simulink model "North_Country_Grid_2024a"  (R2024a)
settings: Solver=VariableStepAuto  StartTime=0.0  StopTime=10  RelTol=1e-3
PreLoadFcn:
  | Ts=50e-6;
InitFcn:
  | xInitial = WindFarmType4AverageModelInit;
  | Ts=50e-6;
undefined symbols (not defined in the file or in its folder): D1, D11, Delta, DiscIntNeverNeededParam, find_system, Fnom_I, Fnom_R, Idc_nom, lagging, level, pulse, test_alpha, Vdc_nom, VLL_nom_I, VLL_nom_R
libraries: spsSecondOrderFilterLib x47, powerlib_extras x38, simulink x34, spsThreePhaseVIMeasurementLib x30, spsFirstOrderFilterLib x29, simulink_extras x26, spsabctodq0Lib x25, spsThreePhaseTransformerTwoWindingsLib x19, spsThreePhaseBreakerLib x18, spsThreePhasePISectionLineLib x17, spsControlledVoltageSourceLib x15, spsOnDelayLib x12
(part 7 of 18)

== system North_Country_Grid_2024a/Noble Chateauguay (Type 4, 106.5 MW)/Wind Farm/Inverter and DC-DC Converter Average Models ==
  note: Pac=Vab*Ia -Vbc*Ic
      | Pdc=Vdc*Idc
  note: Vab Vbc Inverter
      | Average Model
  note: DC-DC Converter
      | Average Model
  note: Inverter and DC-DC Boost Converter
      | Average Models
  note: Current of the boost converter diode
      | This diode is not illustrated in the average model
  IL : Inport
  Iabc_grid_conv : Inport  Port=2
  Uctrl_inverter : Inport  Port=3
  Duty_Cycle : Inport  Port=4
  0.1 : Gain  Gain=0.5
  0.2 : Gain  Gain=-1
  0.5 : Gain  Gain=0.5
  1/C : Gain  Gain=1/C_DClink
  Constant2 : Constant
  Demux : Demux  Outputs=3
  Demux2 : Demux  Outputs=3
  Discrete-Time Integrator : DiscreteIntegrator  InitialCondition=Vdc_nom  SampleTime=Ts  LimitOutput=on  LowerSaturationLimit=eps  ICPrevOutput=DiscIntNeverNeededParam  ICPrevScaledInput=DiscIntNeverNeededParam
  Product{1..4,6..7} (6 alike) : Product  RndMeth=Zero
  Product5 : Product  Inputs=*/  RndMeth=Zero
  Saturation Dynamic : simulink/Discontinuities/Saturation Dynamic  OutMin=[]  OutMax=[]  OutDataTypeStr=Inherit: Same as second input  OutDataType=sfix(16)  OutScaling=2^-10  DoSatur=off
  Saturation Dynamic1 : simulink/Discontinuities/Saturation Dynamic  OutMin=[]  OutMax=[]  OutDataTypeStr=Inherit: Same as second input  OutDataType=sfix(16)  OutScaling=2^-10  DoSatur=off
  Subtract1 : Sum  Inputs=+-
  Subtract2 : Sum  Inputs=+-
  Subtract3 : Sum  Inputs=+-
  Subtract4 : Sum
  Sum : Sum  Inputs=|+-
  Terminator : Terminator
  pu->A : Gain  Gain=Pnom/(3*sqrt(2)/pi*Vnom_gen)  SaturateOnIntegerOverflow=on  OutDataTypeStr=Inherit: Same as input  ParamDataTypeStr=Inherit: Same as input
  "pu->A " : Gain  Gain=Pnom/sqrt(3)/Vnom*sqrt(2)  SaturateOnIntegerOverflow=on  OutDataTypeStr=Inherit: Same as input  ParamDataTypeStr=Inherit: Same as input
  Vab (V) : Outport  VectorParamsAs1DForOutWhenUnconnected=off
  Vbc (V) : Outport  Port=2  VectorParamsAs1DForOutWhenUnconnected=off
  Vswitch (V) : Outport  Port=3  VectorParamsAs1DForOutWhenUnconnected=off
  Vdc (V) : Outport  Port=4  VectorParamsAs1DForOutWhenUnconnected=off
  wires:
  Product1/1 -> Vswitch (V)/1
  Product2/1 -> [Idiode]
  [Vdc] -> Product1/1
  IL/1 -> pu->A/1
  Sum/1 -> Product2/1, Product1/2
  Constant2/1 -> Sum/1
  1/C/1 -> Discrete-Time Integrator/1
  Discrete-Time Integrator/1 -> Vdc (V)/1, Product5/2, [Vdc]
  Subtract4/1 -> 1/C/1
  Demux/1 -> Product3/2  "Ia"
  "pu->A "/1 -> Demux/1
  Demux/2 -> Terminator/1
  Iabc_grid_conv/1 -> "pu->A "/1
  Duty_Cycle/1 -> Sum/2
  Product4/1 -> Subtract2/2
  Product3/1 -> Subtract2/1
  Subtract2/1 -> Product5/1  "Pac"
  Demux/3 -> Product4/2  "Ic"
  [Vab] -> Product3/1
  [Vbc] -> Product4/1
  Product5/1 -> Subtract4/2  "Idc grid converter"
  [Vdc] -> 0.2/1, Saturation Dynamic1/1, Saturation Dynamic/1, Product6/2, Product7/2
  Subtract1/1 -> Product7/1
  Subtract3/1 -> Product6/1
  Product7/1 -> 0.1/1
  Product6/1 -> 0.5/1
  Demux2/3 -> Subtract1/2
  Demux2/2 -> Subtract3/2, Subtract1/1
  Demux2/1 -> Subtract3/1
  0.5/1 -> Saturation Dynamic/2  "Vab_avg"
  0.1/1 -> Saturation Dynamic1/2  "Vbc_avg"
  0.2/1 -> Saturation Dynamic/3, Saturation Dynamic1/3
  Uctrl_inverter/1 -> Demux2/1
  Saturation Dynamic/1 -> Vab (V)/1, [Vab]
  Saturation Dynamic1/1 -> Vbc (V)/1, [Vbc]
  [Idiode] -> Subtract4/1  "Idiode"
  pu->A/1 -> Product2/2

== system North_Country_Grid_2024a/Noble Chateauguay (Type 4, 106.5 MW)/Wind Farm/Wind Turbine ==
  W_wt (pu) : Inport
  Pitch angle (deg) : Inport  Port=2
  Wind speed (m/s) : Inport  Port=3
  ->pu : Gain  Gain=1/Prated
  Avoid div. by zero : Saturate  UpperLimit=inf  LowerLimit=eps
  "Avoid div. by zero " : Saturate  UpperLimit=inf  LowerLimit=eps
  Fcn1 : Fcn  Expr=K1*u[2]/u[1]
  Fcn2 : Fcn  Expr=c1*(c6*u[1] + (-c4 - c3*(2.5 + u[2]) + c2*(1/(u[1] + c7*(2.5 + u[2])) -c8/(1 + (2.5 + u[2])^3)))/exp(c5*(1/(u[1] + c7*(2.5 + u[2])) - c8/(1 + (2.5 + u[2])^3))))
  "K2*Cp*wind^3 " : Fcn  Expr=K2*u[1]^3*u[2]
  Mux : Mux  Inputs=2
  Mux1 : Mux  Inputs=2
  Mux2 : Mux  Inputs=2
  Product2 : Product  Inputs=*/  InputSameDT=on  SaturateOnIntegerOverflow=on  OutDataTypeStr=Inherit: Same as first input
  Tt (pu) : Outport  VectorParamsAs1DForOutWhenUnconnected=off
  wires:
  ->pu/1 -> Product2/1  "power_pu"
  Product2/1 -> Tt (pu)/1
  Wind speed (m/s)/1 -> Avoid div. by zero/1
  Fcn1/1 -> Mux1/1  "lambda"
  Mux1/1 -> Fcn2/1
  Mux/1 -> Fcn1/1
  Fcn2/1 -> Mux2/2  "Cp"
  Mux2/1 -> "K2*Cp*wind^3 "/1
  Pitch angle (deg)/1 -> Mux1/2
  W_wt (pu)/1 -> "Avoid div. by zero "/1
  Avoid div. by zero/1 -> Mux2/1, Mux/1
  "Avoid div. by zero "/1 -> Mux/2, Product2/2
  "K2*Cp*wind^3 "/1 -> ->pu/1

== system North_Country_Grid_2024a/Noble Clinton (Type 4, 100.5 MW)/Wind Farm/Average Switch Voltage ==
  Vswitch : Inport
  Diode : spsDiodeLib/Diode  Ron=1e-6/Nb_wt  Lon=0  Vf=0  IC=0  UseSnubber=off  Rs=1e5  Cs=inf  Measurements=off
  V : spsControlledVoltageSourceLib/Controlled Voltage Source  Initialize=on  Source_Type=AC  Amplitude=0  Phase=0  Frequency=0  Measurements=None
  + : PMIOPort  Side=Right
  - : PMIOPort  Port=2  Side=Left
  wires:
  Vswitch/1 -> V/1
  connections:
  Diode/RConn1 -- V/RConn1
  +/RConn1 -- Diode/LConn1
  -/RConn1 -- V/LConn1

== system North_Country_Grid_2024a/Noble Clinton (Type 4, 100.5 MW)/Wind Farm/Control ==
  note: Inputs
  note: Grid-Side Converter
      | Control System
  note: Speed Regulator & Pitch Control
  note: Excitation
      | Control system
  Vabc_grid : Inport
  Iabc_grid_conv : Inport  Port=2
  Vabc_LL_stator : Inport  Port=3
  Iabc_stator : Inport  Port=4
  IL : Inport  Port=5
  Vdc : Inport  Port=6
  Qref : Inport  Port=7
  angle_rotor : Inport  Port=8
  wr : Inport  Port=9
  Bus Creator : BusCreator  Inputs=2
  Excitation Control system : Subsystem
  Grid-side converter Control system : Subsystem
  Measurement and Transformation : Subsystem
  Speed & Pitch Control : Subsystem
  Unit Delay{1..4,6..7} (6 alike) : UnitDelay  SampleTime=Ts  HasFrameUpgradeWarning=on
  Uctrl_inverter : Outport  VectorParamsAs1DForOutWhenUnconnected=off
  Duty_Cycle : Outport  Port=2  VectorParamsAs1DForOutWhenUnconnected=off
  Pitch_angle : Outport  Port=3  VectorParamsAs1DForOutWhenUnconnected=off
  Vf : Outport  Port=4  VectorParamsAs1DForOutWhenUnconnected=off
  PQ_pu : Outport  Port=5  VectorParamsAs1DForOutWhenUnconnected=off
  wires:
  Excitation Control system/1(Vf) -> Unit Delay2/1
  Speed & Pitch Control/2(Pitch (deg)) -> Unit Delay4/1
  Measurement and Transformation/7(Qmeas) -> [Qmeas]
  Measurement and Transformation/1(Vdq_grid) -> [Vdq_grid]
  Measurement and Transformation/2(Idq_gc) -> [Idq_gc]
  Measurement and Transformation/6(Pmeas) -> [Pmeas]
  Measurement and Transformation/8(Vmeas) -> [Vmeas]
  Measurement and Transformation/10(w_pu) -> [w_pu]
  [Idq_gc] -> Grid-side converter Control system/1(Idq_gc)
  [w_pu] -> Grid-side converter Control system/2(w_pu)
  [Vdq_grid] -> Grid-side converter Control system/3(Vdq_grid)
  [Vdc_meas] -> Grid-side converter Control system/4(Vdc)
  Measurement and Transformation/5(Vdc_meas) -> [Vdc_meas]
  Measurement and Transformation/11("wr ") -> [wr]
  Measurement and Transformation/12("Qref ") -> [Qref]
  [Qref] -> Grid-side converter Control system/5(Qref)
  [Qmeas] -> Grid-side converter Control system/6(Qmeas)
  [Vmeas] -> Grid-side converter Control system/7(Vmeas)
  [wr] -> Speed & Pitch Control/1(wr)
  [Pmeas] -> Speed & Pitch Control/2(Pmeas)
  Speed & Pitch Control/1(Duty_Cycle) -> Unit Delay1/1
  Measurement and Transformation/4(Flux) -> [Flux]
  [Flux] -> Excitation Control system/1(Flux)
  [wr] -> Excitation Control system/2(wr)
  Vabc_grid/1 -> Measurement and Transformation/1(Vabc_grid)
  Iabc_grid_conv/1 -> Measurement and Transformation/2(Iabc_gc)
  Vabc_LL_stator/1 -> Measurement and Transformation/3(Vabc_LL_s)
  Iabc_stator/1 -> Measurement and Transformation/4(Iabc_s)
  Vdc/1 -> Measurement and Transformation/6(Vdc)
  Qref/1 -> Measurement and Transformation/7(Qref)
  angle_rotor/1 -> Measurement and Transformation/8(angle_rotor)
  wr/1 -> Measurement and Transformation/9(wr)
  Grid-side converter Control system/1(Uctrl_inverter) -> Unit Delay3/1
  [Theta_PLL] -> Grid-side converter Control system/8(Theta_PLL)
  Measurement and Transformation/9(Theta_PLL) -> [Theta_PLL]
  Bus Creator/1 -> PQ_pu/1
  Unit Delay3/1 -> Uctrl_inverter/1
  Unit Delay2/1 -> Vf/1
  Unit Delay1/1 -> Duty_Cycle/1
  Unit Delay4/1 -> Pitch_angle/1
  [Pmeas] -> Unit Delay6/1
  [Qmeas] -> Unit Delay7/1
  Unit Delay6/1 -> Bus Creator/1  "P_pu"
  Unit Delay7/1 -> Bus Creator/2  "Q_pu"
  Measurement and Transformation/3("IL ") -> [IL]
  IL/1 -> Measurement and Transformation/5(IL)
  [IL] -> Speed & Pitch Control/3(IL)

== system North_Country_Grid_2024a/Noble Clinton (Type 4, 100.5 MW)/Wind Farm/Drive Train ==
  note: Wind turbine drive train based on a 2-masse model
  note: Turbine
  note: Shaft
  T_wt (pu) : Inport
  Generator speed (pu) : Inport  Port=2
  1_2H_WT : Gain  Gain=1/(2*H_WT)  SaturateOnIntegerOverflow=on  OutDataTypeStr=Inherit: Same as input  ParamDataTypeStr=Inherit: Same as input
  Discrete-Time Integrator : DiscreteIntegrator  InitialCondition=w_wt0  SampleTime=Ts  ICPrevOutput=DiscIntNeverNeededParam  ICPrevScaledInput=DiscIntNeverNeededParam
  Discrete-Time Integrator1 : DiscreteIntegrator  InitialCondition=torque0/Ksh  SampleTime=Ts  ICPrevOutput=DiscIntNeverNeededParam  ICPrevScaledInput=DiscIntNeverNeededParam
  Mutual damping : Gain  Gain=D_mutual  SaturateOnIntegerOverflow=on  OutDataTypeStr=Inherit: Same as input  ParamDataTypeStr=Inherit: Same as input
  Stiffness : Gain  Gain=Ksh  SaturateOnIntegerOverflow=on  OutDataTypeStr=Inherit: Same as input  ParamDataTypeStr=Inherit: Same as input
  Sum : Sum  Inputs=+-  InputSameDT=on  SaturateOnIntegerOverflow=on  OutDataTypeStr=Inherit: Same as first input
  Sum1 : Sum  Inputs=+-  InputSameDT=on  SaturateOnIntegerOverflow=on  OutDataTypeStr=Inherit: Same as first input
  Sum2 : Sum  InputSameDT=on  SaturateOnIntegerOverflow=on  OutDataTypeStr=Inherit: Same as first input
  wbase : Gain  Gain=wbase  SaturateOnIntegerOverflow=on  OutDataTypeStr=Inherit: Same as input  ParamDataTypeStr=Inherit: Same as input
  W_wt (pu) : Outport  VectorParamsAs1DForOutWhenUnconnected=off
  T_shaft (pu) : Outport  Port=2  VectorParamsAs1DForOutWhenUnconnected=off
  wires:
  T_wt (pu)/1 -> Sum/1
  Sum2/1 -> T_shaft (pu)/1, Sum/2
  Mutual damping/1 -> Sum2/2
  Sum1/1 -> Mutual damping/1, wbase/1
  Generator speed (pu)/1 -> Sum1/2
  Discrete-Time Integrator/1 -> W_wt (pu)/1, Sum1/1
  1_2H_WT/1 -> Discrete-Time Integrator/1
  Sum/1 -> 1_2H_WT/1
  Stiffness/1 -> Sum2/1
  Discrete-Time Integrator1/1 -> Stiffness/1
  wbase/1 -> Discrete-Time Integrator1/1

== system North_Country_Grid_2024a/Noble Clinton (Type 4, 100.5 MW)/Wind Farm/Inverter and DC-DC Converter Average Models ==
  note: Pac=Vab*Ia -Vbc*Ic
      | Pdc=Vdc*Idc
  note: Vab Vbc Inverter
      | Average Model
  note: DC-DC Converter
      | Average Model
  note: Inverter and DC-DC Boost Converter
      | Average Models
  note: Current of the boost converter diode
      | This diode is not illustrated in the average model
  IL : Inport
  Iabc_grid_conv : Inport  Port=2
  Uctrl_inverter : Inport  Port=3
  Duty_Cycle : Inport  Port=4
  0.1 : Gain  Gain=0.5
  0.2 : Gain  Gain=-1
  0.5 : Gain  Gain=0.5
  1/C : Gain  Gain=1/C_DClink
  Constant2 : Constant
  Demux : Demux  Outputs=3
  Demux2 : Demux  Outputs=3
  Discrete-Time Integrator : DiscreteIntegrator  InitialCondition=Vdc_nom  SampleTime=Ts  LimitOutput=on  LowerSaturationLimit=eps  ICPrevOutput=DiscIntNeverNeededParam  ICPrevScaledInput=DiscIntNeverNeededParam
  Product{1..4,6..7} (6 alike) : Product  RndMeth=Zero
  Product5 : Product  Inputs=*/  RndMeth=Zero
  Saturation Dynamic : simulink/Discontinuities/Saturation Dynamic  OutMin=[]  OutMax=[]  OutDataTypeStr=Inherit: Same as second input  OutDataType=sfix(16)  OutScaling=2^-10  DoSatur=off
  Saturation Dynamic1 : simulink/Discontinuities/Saturation Dynamic  OutMin=[]  OutMax=[]  OutDataTypeStr=Inherit: Same as second input  OutDataType=sfix(16)  OutScaling=2^-10  DoSatur=off
  Subtract1 : Sum  Inputs=+-
  Subtract2 : Sum  Inputs=+-
  Subtract3 : Sum  Inputs=+-
  Subtract4 : Sum
  Sum : Sum  Inputs=|+-
  Terminator : Terminator
  pu->A : Gain  Gain=Pnom/(3*sqrt(2)/pi*Vnom_gen)  SaturateOnIntegerOverflow=on  OutDataTypeStr=Inherit: Same as input  ParamDataTypeStr=Inherit: Same as input
  "pu->A " : Gain  Gain=Pnom/sqrt(3)/Vnom*sqrt(2)  SaturateOnIntegerOverflow=on  OutDataTypeStr=Inherit: Same as input  ParamDataTypeStr=Inherit: Same as input
  Vab (V) : Outport  VectorParamsAs1DForOutWhenUnconnected=off
  Vbc (V) : Outport  Port=2  VectorParamsAs1DForOutWhenUnconnected=off
  Vswitch (V) : Outport  Port=3  VectorParamsAs1DForOutWhenUnconnected=off
  Vdc (V) : Outport  Port=4  VectorParamsAs1DForOutWhenUnconnected=off
  wires:
  Product1/1 -> Vswitch (V)/1
  Product2/1 -> [Idiode]
  [Vdc] -> Product1/1
  IL/1 -> pu->A/1
  Sum/1 -> Product2/1, Product1/2
  Constant2/1 -> Sum/1
  1/C/1 -> Discrete-Time Integrator/1
  Discrete-Time Integrator/1 -> Vdc (V)/1, Product5/2, [Vdc]
  Subtract4/1 -> 1/C/1
  Demux/1 -> Product3/2  "Ia"
  "pu->A "/1 -> Demux/1
  Demux/2 -> Terminator/1
  Iabc_grid_conv/1 -> "pu->A "/1
  Duty_Cycle/1 -> Sum/2
  Product4/1 -> Subtract2/2
  Product3/1 -> Subtract2/1
  Subtract2/1 -> Product5/1  "Pac"
  Demux/3 -> Product4/2  "Ic"
  [Vab] -> Product3/1
  [Vbc] -> Product4/1
  Product5/1 -> Subtract4/2  "Idc grid converter"
  [Vdc] -> 0.2/1, Saturation Dynamic1/1, Saturation Dynamic/1, Product6/2, Product7/2
  Subtract1/1 -> Product7/1
  Subtract3/1 -> Product6/1
  Product7/1 -> 0.1/1
  Product6/1 -> 0.5/1
  Demux2/3 -> Subtract1/2
  Demux2/2 -> Subtract3/2, Subtract1/1
  Demux2/1 -> Subtract3/1
  0.5/1 -> Saturation Dynamic/2  "Vab_avg"
  0.1/1 -> Saturation Dynamic1/2  "Vbc_avg"
  0.2/1 -> Saturation Dynamic/3, Saturation Dynamic1/3
  Uctrl_inverter/1 -> Demux2/1
  Saturation Dynamic/1 -> Vab (V)/1, [Vab]
  Saturation Dynamic1/1 -> Vbc (V)/1, [Vbc]
  [Idiode] -> Subtract4/1  "Idiode"
  pu->A/1 -> Product2/2

== system North_Country_Grid_2024a/Noble Clinton (Type 4, 100.5 MW)/Wind Farm/Wind Turbine ==
  W_wt (pu) : Inport
  Pitch angle (deg) : Inport  Port=2
  Wind speed (m/s) : Inport  Port=3
  ->pu : Gain  Gain=1/Prated
  Avoid div. by zero : Saturate  UpperLimit=inf  LowerLimit=eps
  "Avoid div. by zero " : Saturate  UpperLimit=inf  LowerLimit=eps
  Fcn1 : Fcn  Expr=K1*u[2]/u[1]
  Fcn2 : Fcn  Expr=c1*(c6*u[1] + (-c4 - c3*(2.5 + u[2]) + c2*(1/(u[1] + c7*(2.5 + u[2])) -c8/(1 + (2.5 + u[2])^3)))/exp(c5*(1/(u[1] + c7*(2.5 + u[2])) - c8/(1 + (2.5 + u[2])^3))))
  "K2*Cp*wind^3 " : Fcn  Expr=K2*u[1]^3*u[2]
  Mux : Mux  Inputs=2
  Mux1 : Mux  Inputs=2
  Mux2 : Mux  Inputs=2
  Product2 : Product  Inputs=*/  InputSameDT=on  SaturateOnIntegerOverflow=on  OutDataTypeStr=Inherit: Same as first input
  Tt (pu) : Outport  VectorParamsAs1DForOutWhenUnconnected=off
  wires:
  ->pu/1 -> Product2/1  "power_pu"
  Product2/1 -> Tt (pu)/1
  Wind speed (m/s)/1 -> Avoid div. by zero/1
  Fcn1/1 -> Mux1/1  "lambda"
  Mux1/1 -> Fcn2/1
  Mux/1 -> Fcn1/1
  Fcn2/1 -> Mux2/2  "Cp"
  Mux2/1 -> "K2*Cp*wind^3 "/1
  Pitch angle (deg)/1 -> Mux1/2
  W_wt (pu)/1 -> "Avoid div. by zero "/1
  Avoid div. by zero/1 -> Mux2/1, Mux/1
  "Avoid div. by zero "/1 -> Mux/2, Product2/2
  "K2*Cp*wind^3 "/1 -> ->pu/1

== system North_Country_Grid_2024a/Noble Ellenburg (Type 4, 81 MW)/Wind Farm/Average Switch Voltage ==
  Vswitch : Inport
  Diode : spsDiodeLib/Diode  Ron=1e-6/Nb_wt  Lon=0  Vf=0  IC=0  UseSnubber=off  Rs=1e5  Cs=inf  Measurements=off
  V : spsControlledVoltageSourceLib/Controlled Voltage Source  Initialize=on  Source_Type=AC  Amplitude=0  Phase=0  Frequency=0  Measurements=None
  + : PMIOPort  Side=Right
  - : PMIOPort  Port=2  Side=Left
  wires:
  Vswitch/1 -> V/1
  connections:
  Diode/RConn1 -- V/RConn1
  +/RConn1 -- Diode/LConn1
  -/RConn1 -- V/LConn1

== system North_Country_Grid_2024a/Noble Ellenburg (Type 4, 81 MW)/Wind Farm/Control ==
  note: Inputs
  note: Grid-Side Converter
      | Control System
  note: Speed Regulator & Pitch Control
  note: Excitation
      | Control system
  Vabc_grid : Inport
  Iabc_grid_conv : Inport  Port=2
  Vabc_LL_stator : Inport  Port=3
  Iabc_stator : Inport  Port=4
  IL : Inport  Port=5
  Vdc : Inport  Port=6
  Qref : Inport  Port=7
  angle_rotor : Inport  Port=8
  wr : Inport  Port=9
  Bus Creator : BusCreator  Inputs=2
  Excitation Control system : Subsystem
  Grid-side converter Control system : Subsystem
  Measurement and Transformation : Subsystem
  Speed & Pitch Control : Subsystem
  Unit Delay{1..4,6..7} (6 alike) : UnitDelay  SampleTime=Ts  HasFrameUpgradeWarning=on
  Uctrl_inverter : Outport  VectorParamsAs1DForOutWhenUnconnected=off
  Duty_Cycle : Outport  Port=2  VectorParamsAs1DForOutWhenUnconnected=off
  Pitch_angle : Outport  Port=3  VectorParamsAs1DForOutWhenUnconnected=off
  Vf : Outport  Port=4  VectorParamsAs1DForOutWhenUnconnected=off
  PQ_pu : Outport  Port=5  VectorParamsAs1DForOutWhenUnconnected=off
  wires:
  Excitation Control system/1(Vf) -> Unit Delay2/1
  Speed & Pitch Control/2(Pitch (deg)) -> Unit Delay4/1
  Measurement and Transformation/7(Qmeas) -> [Qmeas]
  Measurement and Transformation/1(Vdq_grid) -> [Vdq_grid]
  Measurement and Transformation/2(Idq_gc) -> [Idq_gc]
  Measurement and Transformation/6(Pmeas) -> [Pmeas]
  Measurement and Transformation/8(Vmeas) -> [Vmeas]
  Measurement and Transformation/10(w_pu) -> [w_pu]
  [Idq_gc] -> Grid-side converter Control system/1(Idq_gc)
  [w_pu] -> Grid-side converter Control system/2(w_pu)
  [Vdq_grid] -> Grid-side converter Control system/3(Vdq_grid)
  [Vdc_meas] -> Grid-side converter Control system/4(Vdc)
  Measurement and Transformation/5(Vdc_meas) -> [Vdc_meas]
  Measurement and Transformation/11("wr ") -> [wr]
  Measurement and Transformation/12("Qref ") -> [Qref]
  [Qref] -> Grid-side converter Control system/5(Qref)
  [Qmeas] -> Grid-side converter Control system/6(Qmeas)
  [Vmeas] -> Grid-side converter Control system/7(Vmeas)
  [wr] -> Speed & Pitch Control/1(wr)
  [Pmeas] -> Speed & Pitch Control/2(Pmeas)
  Speed & Pitch Control/1(Duty_Cycle) -> Unit Delay1/1
  Measurement and Transformation/4(Flux) -> [Flux]
  [Flux] -> Excitation Control system/1(Flux)
  [wr] -> Excitation Control system/2(wr)
  Vabc_grid/1 -> Measurement and Transformation/1(Vabc_grid)
  Iabc_grid_conv/1 -> Measurement and Transformation/2(Iabc_gc)
  Vabc_LL_stator/1 -> Measurement and Transformation/3(Vabc_LL_s)
  Iabc_stator/1 -> Measurement and Transformation/4(Iabc_s)
  Vdc/1 -> Measurement and Transformation/6(Vdc)
  Qref/1 -> Measurement and Transformation/7(Qref)
  angle_rotor/1 -> Measurement and Transformation/8(angle_rotor)
  wr/1 -> Measurement and Transformation/9(wr)
  Grid-side converter Control system/1(Uctrl_inverter) -> Unit Delay3/1
  [Theta_PLL] -> Grid-side converter Control system/8(Theta_PLL)
  Measurement and Transformation/9(Theta_PLL) -> [Theta_PLL]
  Bus Creator/1 -> PQ_pu/1
  Unit Delay3/1 -> Uctrl_inverter/1
  Unit Delay2/1 -> Vf/1
  Unit Delay1/1 -> Duty_Cycle/1
  Unit Delay4/1 -> Pitch_angle/1
  [Pmeas] -> Unit Delay6/1
  [Qmeas] -> Unit Delay7/1
  Unit Delay6/1 -> Bus Creator/1  "P_pu"
  Unit Delay7/1 -> Bus Creator/2  "Q_pu"
  Measurement and Transformation/3("IL ") -> [IL]
  IL/1 -> Measurement and Transformation/5(IL)
  [IL] -> Speed & Pitch Control/3(IL)

== system North_Country_Grid_2024a/Noble Ellenburg (Type 4, 81 MW)/Wind Farm/Drive Train ==
  note: Wind turbine drive train based on a 2-masse model
  note: Turbine
  note: Shaft
  T_wt (pu) : Inport
  Generator speed (pu) : Inport  Port=2
  1_2H_WT : Gain  Gain=1/(2*H_WT)  SaturateOnIntegerOverflow=on  OutDataTypeStr=Inherit: Same as input  ParamDataTypeStr=Inherit: Same as input
  Discrete-Time Integrator : DiscreteIntegrator  InitialCondition=w_wt0  SampleTime=Ts  ICPrevOutput=DiscIntNeverNeededParam  ICPrevScaledInput=DiscIntNeverNeededParam
  Discrete-Time Integrator1 : DiscreteIntegrator  InitialCondition=torque0/Ksh  SampleTime=Ts  ICPrevOutput=DiscIntNeverNeededParam  ICPrevScaledInput=DiscIntNeverNeededParam
  Mutual damping : Gain  Gain=D_mutual  SaturateOnIntegerOverflow=on  OutDataTypeStr=Inherit: Same as input  ParamDataTypeStr=Inherit: Same as input
  Stiffness : Gain  Gain=Ksh  SaturateOnIntegerOverflow=on  OutDataTypeStr=Inherit: Same as input  ParamDataTypeStr=Inherit: Same as input
  Sum : Sum  Inputs=+-  InputSameDT=on  SaturateOnIntegerOverflow=on  OutDataTypeStr=Inherit: Same as first input
  Sum1 : Sum  Inputs=+-  InputSameDT=on  SaturateOnIntegerOverflow=on  OutDataTypeStr=Inherit: Same as first input
  Sum2 : Sum  InputSameDT=on  SaturateOnIntegerOverflow=on  OutDataTypeStr=Inherit: Same as first input
  wbase : Gain  Gain=wbase  SaturateOnIntegerOverflow=on  OutDataTypeStr=Inherit: Same as input  ParamDataTypeStr=Inherit: Same as input
  W_wt (pu) : Outport  VectorParamsAs1DForOutWhenUnconnected=off
  T_shaft (pu) : Outport  Port=2  VectorParamsAs1DForOutWhenUnconnected=off
  wires:
  T_wt (pu)/1 -> Sum/1
  Sum2/1 -> T_shaft (pu)/1, Sum/2
  Mutual damping/1 -> Sum2/2
  Sum1/1 -> Mutual damping/1, wbase/1
  Generator speed (pu)/1 -> Sum1/2
  Discrete-Time Integrator/1 -> W_wt (pu)/1, Sum1/1
  1_2H_WT/1 -> Discrete-Time Integrator/1
  Sum/1 -> 1_2H_WT/1
  Stiffness/1 -> Sum2/1
  Discrete-Time Integrator1/1 -> Stiffness/1
  wbase/1 -> Discrete-Time Integrator1/1

== system North_Country_Grid_2024a/Noble Ellenburg (Type 4, 81 MW)/Wind Farm/Inverter and DC-DC Converter Average Models ==
  note: Pac=Vab*Ia -Vbc*Ic
      | Pdc=Vdc*Idc
  note: Vab Vbc Inverter
      | Average Model
  note: DC-DC Converter
      | Average Model
  note: Inverter and DC-DC Boost Converter
      | Average Models
  note: Current of the boost converter diode
      | This diode is not illustrated in the average model
  IL : Inport
  Iabc_grid_conv : Inport  Port=2
  Uctrl_inverter : Inport  Port=3
  Duty_Cycle : Inport  Port=4
  0.1 : Gain  Gain=0.5
  0.2 : Gain  Gain=-1
  0.5 : Gain  Gain=0.5
  1/C : Gain  Gain=1/C_DClink
  Constant2 : Constant
  Demux : Demux  Outputs=3
  Demux2 : Demux  Outputs=3
  Discrete-Time Integrator : DiscreteIntegrator  InitialCondition=Vdc_nom  SampleTime=Ts  LimitOutput=on  LowerSaturationLimit=eps  ICPrevOutput=DiscIntNeverNeededParam  ICPrevScaledInput=DiscIntNeverNeededParam
  Product{1..4,6..7} (6 alike) : Product  RndMeth=Zero
  Product5 : Product  Inputs=*/  RndMeth=Zero
  Saturation Dynamic : simulink/Discontinuities/Saturation Dynamic  OutMin=[]  OutMax=[]  OutDataTypeStr=Inherit: Same as second input  OutDataType=sfix(16)  OutScaling=2^-10  DoSatur=off
  Saturation Dynamic1 : simulink/Discontinuities/Saturation Dynamic  OutMin=[]  OutMax=[]  OutDataTypeStr=Inherit: Same as second input  OutDataType=sfix(16)  OutScaling=2^-10  DoSatur=off
  Subtract1 : Sum  Inputs=+-
  Subtract2 : Sum  Inputs=+-
  Subtract3 : Sum  Inputs=+-
  Subtract4 : Sum
  Sum : Sum  Inputs=|+-
  Terminator : Terminator
  pu->A : Gain  Gain=Pnom/(3*sqrt(2)/pi*Vnom_gen)  SaturateOnIntegerOverflow=on  OutDataTypeStr=Inherit: Same as input  ParamDataTypeStr=Inherit: Same as input
  "pu->A " : Gain  Gain=Pnom/sqrt(3)/Vnom*sqrt(2)  SaturateOnIntegerOverflow=on  OutDataTypeStr=Inherit: Same as input  ParamDataTypeStr=Inherit: Same as input
  Vab (V) : Outport  VectorParamsAs1DForOutWhenUnconnected=off
  Vbc (V) : Outport  Port=2  VectorParamsAs1DForOutWhenUnconnected=off
  Vswitch (V) : Outport  Port=3  VectorParamsAs1DForOutWhenUnconnected=off
  Vdc (V) : Outport  Port=4  VectorParamsAs1DForOutWhenUnconnected=off
  wires:
  Product1/1 -> Vswitch (V)/1
  Product2/1 -> [Idiode]
  [Vdc] -> Product1/1
  IL/1 -> pu->A/1
  Sum/1 -> Product2/1, Product1/2
  Constant2/1 -> Sum/1
  1/C/1 -> Discrete-Time Integrator/1
  Discrete-Time Integrator/1 -> Vdc (V)/1, Product5/2, [Vdc]
  Subtract4/1 -> 1/C/1
  Demux/1 -> Product3/2  "Ia"
  "pu->A "/1 -> Demux/1
  Demux/2 -> Terminator/1
  Iabc_grid_conv/1 -> "pu->A "/1
  Duty_Cycle/1 -> Sum/2
  Product4/1 -> Subtract2/2
  Product3/1 -> Subtract2/1
  Subtract2/1 -> Product5/1  "Pac"
  Demux/3 -> Product4/2  "Ic"
  [Vab] -> Product3/1
  [Vbc] -> Product4/1
  Product5/1 -> Subtract4/2  "Idc grid converter"
  [Vdc] -> 0.2/1, Saturation Dynamic1/1, Saturation Dynamic/1, Product6/2, Product7/2
  Subtract1/1 -> Product7/1
  Subtract3/1 -> Product6/1
  Product7/1 -> 0.1/1
  Product6/1 -> 0.5/1
  Demux2/3 -> Subtract1/2
  Demux2/2 -> Subtract3/2, Subtract1/1
  Demux2/1 -> Subtract3/1
  0.5/1 -> Saturation Dynamic/2  "Vab_avg"
  0.1/1 -> Saturation Dynamic1/2  "Vbc_avg"
  0.2/1 -> Saturation Dynamic/3, Saturation Dynamic1/3
  Uctrl_inverter/1 -> Demux2/1
  Saturation Dynamic/1 -> Vab (V)/1, [Vab]
  Saturation Dynamic1/1 -> Vbc (V)/1, [Vbc]
  [Idiode] -> Subtract4/1  "Idiode"
  pu->A/1 -> Product2/2

== system North_Country_Grid_2024a/Noble Ellenburg (Type 4, 81 MW)/Wind Farm/Wind Turbine ==
  W_wt (pu) : Inport
  Pitch angle (deg) : Inport  Port=2
  Wind speed (m/s) : Inport  Port=3
  ->pu : Gain  Gain=1/Prated
  Avoid div. by zero : Saturate  UpperLimit=inf  LowerLimit=eps
  "Avoid div. by zero " : Saturate  UpperLimit=inf  LowerLimit=eps
  Fcn1 : Fcn  Expr=K1*u[2]/u[1]
  Fcn2 : Fcn  Expr=c1*(c6*u[1] + (-c4 - c3*(2.5 + u[2]) + c2*(1/(u[1] + c7*(2.5 + u[2])) -c8/(1 + (2.5 + u[2])^3)))/exp(c5*(1/(u[1] + c7*(2.5 + u[2])) - c8/(1 + (2.5 + u[2])^3))))
  "K2*Cp*wind^3 " : Fcn  Expr=K2*u[1]^3*u[2]
  Mux : Mux  Inputs=2
  Mux1 : Mux  Inputs=2
  Mux2 : Mux  Inputs=2
  Product2 : Product  Inputs=*/  InputSameDT=on  SaturateOnIntegerOverflow=on  OutDataTypeStr=Inherit: Same as first input
  Tt (pu) : Outport  VectorParamsAs1DForOutWhenUnconnected=off
  wires:
  ->pu/1 -> Product2/1  "power_pu"
  Product2/1 -> Tt (pu)/1
  Wind speed (m/s)/1 -> Avoid div. by zero/1
  Fcn1/1 -> Mux1/1  "lambda"
  Mux1/1 -> Fcn2/1
  Mux/1 -> Fcn1/1
  Fcn2/1 -> Mux2/2  "Cp"
  Mux2/1 -> "K2*Cp*wind^3 "/1
  Pitch angle (deg)/1 -> Mux1/2
  W_wt (pu)/1 -> "Avoid div. by zero "/1
  Avoid div. by zero/1 -> Mux2/1, Mux/1
  "Avoid div. by zero "/1 -> Mux/2, Product2/2
  "K2*Cp*wind^3 "/1 -> ->pu/1

== system North_Country_Grid_2024a/Chateauguay HVDC Back-to-Back Converter/Inverter Control and Protection/Gamma Measurement/Gamma Measurement (D1 bridge) ==
  note: Outgoing  Conducting      Commutation Voltage (Uak)
      | Valve         Valves                Y          D1(lag)     D11(lead)
      | ---------      ----------------     --------   ------------    -------------
      |     1                 2-3                Uab         Ua              -Ub
      |     2                 3-4                Uac        -Uc                Ua
      |     3                 4-5                Ubc         Ub              -Uc
      |     4                 5-6                Uba       -Ua                Ub
      |     5                 6-1                Uca         Uc              -Ua
      |     6                 1-2                Ucb        -Ub               Uc
  note: Linear interpolation for
      | zero crossing detection error
      |  in a discete system
  note: Gamma measurement of a six-pulse thyristor bridge
  note: Silvano Casoria
      | Power Systems and Mathematics
      |  IREQ, Hydro-Quebec
  I_th(1-6) : Inport  PortDimensions=6
  Uabc : Inport  Port=2  PortDimensions=3
  Freq : Inport  Port=3
  Pulses(1-6) : Inport  Port=4  PortDimensions=6
  Bistable : spsBistableLib/Bistable  Qpriority=Set  ic=0  Ts=Ts
  Clock : Clock
  Commutation Voltages : Subsystem
  Constant : Constant  Value=InterpolationOn
  Divide1 : Product  Inputs=**
  Edge Detector_1 : spsEdgeDetectorLib/Edge Detector  model=Rising  ic=0  Ts=Ts
  Edge Detector_2 : spsEdgeDetectorLib/Edge Detector  model=Rising  ic=0  Ts=Ts
  Gain1 : Gain  Gain=1/6  SaturateOnIntegerOverflow=on  OutDataTypeStr=Inherit: Same as input  ParamDataTypeStr=Inherit: Same as input
  Gain2 : Gain  Gain=360  SaturateOnIntegerOverflow=on  OutDataTypeStr=Inherit: Same as input  ParamDataTypeStr=Inherit: Same as input
  Gain7 : Gain  Gain=-1  SaturateOnIntegerOverflow=on  OutDataTypeStr=Inherit: Same as input  ParamDataTypeStr=Inherit: Same as input
  Hit (Falling) : HitCross  HitCrossingOffset=Ith_min  HitCrossingDirection=falling  SampleTime=Ts
  "Hit (Falling) " : HitCross  HitCrossingDirection=falling  SampleTime=Ts
  Logical Operator1 : Logic  AllPortsSameDT=off  OutDataTypeStr=boolean
  Logical Operator2 : Logic  Operator=NOT  AllPortsSameDT=off  OutDataTypeStr=boolean
  MinMax1 : MinMax  InputSameDT=on  SaturateOnIntegerOverflow=on
  Monostable_1 (4 deg) : spsMonostableLib/Monostable  EdgeDetect=Rising  PulseDuration=4/(360*f0)  ic=0  Ts=Ts
  Monostable_2 (86 deg) : spsMonostableLib/Monostable  EdgeDetect=Rising  PulseDuration=86/(360*f0)  ic=0  Ts=Ts
  Product1 : Product  SaturateOnIntegerOverflow=on  OutDataTypeStr=Inherit: Same as first input
  Pulse_counter_sampler (1-6) : Subsystem  TreatAsAtomicUnit=on
  Sample and Hold_1 : spsSampleandHoldLib/Sample and Hold  ic=0  Ts=Ts
  Sample and Hold_2 : spsSampleandHoldLib/Sample and Hold  ic=0  Ts=Ts
  Sample and Hold_3 : spsSampleandHoldLib/Sample and Hold  ic=0  Ts=Ts
  Subtract1 : Sum  Inputs=+-
  Sum : Sum  Inputs=|-+  InputSameDT=on  SaturateOnIntegerOverflow=on  OutDataTypeStr=Inherit: Same as first input
  Sum1 : Sum  Inputs=+  InputSameDT=on  SaturateOnIntegerOverflow=on  OutDataTypeStr=Inherit: Same as first input
  Terminator2 : Terminator
  Zero crossing interpolation : Subsystem  mask(Discrete - Hit crossing time interval error calculation by linear interpolation){y0=0, TOL=V_tol, Ts=Ts}
      mask prompts: y0 "Hit crossing offset (y0):"; TOL "Tolerance:"; Ts "Sample time:"
      mask help:
      | The function calculates, using the linear interpolation,an approximation of the time interval error in detencting when the input signal  (y) crosses (in any direction)the offset value "y0".
      | The output (t_err) is the time interval error which value is between 0 and the sample time. The calculation is done (otherwise t_err = 0) if the input signal changes by more then the value defined by the parameter "Tolerance".
      | This change is measured during the time step when the hit crossing takes place.
  gamma_min (deg) : Outport  VectorParamsAs1DForOutWhenUnconnected=off
  gamma_mean (deg) : Outport  Port=2  VectorParamsAs1DForOutWhenUnconnected=off
  Ucom(1-6) : Outport  Port=3  VectorParamsAs1DForOutWhenUnconnected=off
  gamma (deg) : Outport  Port=4  VectorParamsAs1DForOutWhenUnconnected=off
  wires:
  Divide1/1 -> Subtract1/2
  Pulse_counter_sampler (1-6)/2(pulse_n) -> Terminator2/1
  MinMax1/1 -> gamma_min (deg)/1
  Gain1/1 -> gamma_mean (deg)/1
  Sum1/1 -> Gain1/1
  Pulse_counter_sampler (1-6)/1(angle) -> gamma (deg)/1
  Sample and Hold_3/1 -> Product1/1  "t_gamma"
  Subtract1/1 -> Sum/2  "t1"
  Sample and Hold_1/1 -> Sum/1  "t0"
  Gain2/1 -> Product1/2
  Freq/1 -> Gain2/1
  Uabc/1 -> Commutation Voltages/1(Uabc)  "Ua Ub Uc"
  Commutation Voltages/1(Ucom (1-6)) -> Gain7/1, Zero crossing interpolation/1(y), Ucom(1-6)/1
  Gain7/1 -> "Hit (Falling) "/1
  Monostable_1 (4 deg)/1 -> Bistable/1
  "Hit (Falling) "/1 -> Monostable_2 (86 deg)/1
  Sum/1 -> Sample and Hold_3/1
  Product1/1 -> MinMax1/1, Sum1/1, Pulse_counter_sampler (1-6)/1(angles(1-6))  "gamma(1_6)"
  Edge Detector_2/1 -> Sample and Hold_2/2, Sample and Hold_3/2, Zero crossing interpolation/2(Sample)
  Pulses(1-6)/1 -> Pulse_counter_sampler (1-6)/Trigger, Logical Operator2/1
  Logical Operator2/1 -> Logical Operator1/2
  I_th(1-6)/1 -> Hit (Falling)/1
  Logical Operator1/1 -> Monostable_1 (4 deg)/1
  Hit (Falling)/1 -> Logical Operator1/1
  Constant/1 -> Zero crossing interpolation/Enable, Divide1/1
  Clock/1 -> Sample and Hold_2/1, Sample and Hold_1/1
  Zero crossing interpolation/1(t_err) -> Divide1/2  "correction"
  Bistable/1 -> Edge Detector_1/1
  Monostable_2 (86 deg)/1 -> Bistable/2
  Bistable/2 -> Edge Detector_2/1
  Edge Detector_1/1 -> Sample and Hold_1/2
  Sample and Hold_2/1 -> Subtract1/1  "t1_tmp"

== system North_Country_Grid_2024a/Chateauguay HVDC Back-to-Back Converter/Inverter Control and Protection/Gamma Measurement/Gamma Measurement (Y bridge) ==
  note: Outgoing  Conducting      Commutation Voltage (Uak)
      | Valve         Valves                Y          D1(lag)     D11(lead)
      | ---------      ----------------     --------   ------------    -------------
      |     1                 2-3                Uab         Ua              -Ub
      |     2                 3-4                Uac        -Uc                Ua
      |     3                 4-5                Ubc         Ub              -Uc
      |     4                 5-6                Uba       -Ua                Ub
      |     5                 6-1                Uca         Uc              -Ua
      |     6                 1-2                Ucb        -Ub               Uc
  note: Linear interpolation for
      | zero crossing detection error
      |  in a discete system
  note: Gamma measurement of a six-pulse thyristor bridge
  note: Silvano Casoria
      | Power Systems and Mathematics
      |  IREQ, Hydro-Quebec
  I_th(1-6) : Inport  PortDimensions=6
  Uabc : Inport  Port=2  PortDimensions=3
  Freq : Inport  Port=3
  Pulses(1-6) : Inport  Port=4  PortDimensions=6
  Bistable : spsBistableLib/Bistable  Qpriority=Set  ic=0  Ts=Ts
  Clock : Clock
  Commutation Voltages : Subsystem
  Constant : Constant  Value=InterpolationOn
  Divide1 : Product  Inputs=**
  Edge Detector_1 : spsEdgeDetectorLib/Edge Detector  model=Rising  ic=0  Ts=Ts
  Edge Detector_2 : spsEdgeDetectorLib/Edge Detector  model=Rising  ic=0  Ts=Ts
  Gain1 : Gain  Gain=1/6  SaturateOnIntegerOverflow=on  OutDataTypeStr=Inherit: Same as input  ParamDataTypeStr=Inherit: Same as input
  Gain2 : Gain  Gain=360  SaturateOnIntegerOverflow=on  OutDataTypeStr=Inherit: Same as input  ParamDataTypeStr=Inherit: Same as input
  Gain7 : Gain  Gain=-1  SaturateOnIntegerOverflow=on  OutDataTypeStr=Inherit: Same as input  ParamDataTypeStr=Inherit: Same as input
  Hit (Falling) : HitCross  HitCrossingOffset=Ith_min  HitCrossingDirection=falling  SampleTime=Ts
  "Hit (Falling) " : HitCross  HitCrossingDirection=falling  SampleTime=Ts
  Logical Operator1 : Logic  AllPortsSameDT=off  OutDataTypeStr=boolean
  Logical Operator2 : Logic  Operator=NOT  AllPortsSameDT=off  OutDataTypeStr=boolean
  MinMax1 : MinMax  InputSameDT=on  SaturateOnIntegerOverflow=on
  Monostable_1 (4 deg) : spsMonostableLib/Monostable  EdgeDetect=Rising  PulseDuration=4/(360*f0)  ic=0  Ts=Ts
  Monostable_2 (86 deg) : spsMonostableLib/Monostable  EdgeDetect=Rising  PulseDuration=86/(360*f0)  ic=0  Ts=Ts
  Product1 : Product  SaturateOnIntegerOverflow=on  OutDataTypeStr=Inherit: Same as first input
  Pulse_counter_sampler (1-6) : Subsystem  TreatAsAtomicUnit=on
  Sample and Hold_1 : spsSampleandHoldLib/Sample and Hold  ic=0  Ts=Ts
  Sample and Hold_2 : spsSampleandHoldLib/Sample and Hold  ic=0  Ts=Ts
  Sample and Hold_3 : spsSampleandHoldLib/Sample and Hold  ic=0  Ts=Ts
  Subtract1 : Sum  Inputs=+-
  Sum : Sum  Inputs=|-+  InputSameDT=on  SaturateOnIntegerOverflow=on  OutDataTypeStr=Inherit: Same as first input
  Sum1 : Sum  Inputs=+  InputSameDT=on  SaturateOnIntegerOverflow=on  OutDataTypeStr=Inherit: Same as first input
  Terminator2 : Terminator
  Zero crossing interpolation : Subsystem  mask(Discrete - Hit crossing time interval error calculation by linear interpolation){y0=0, TOL=V_tol, Ts=Ts}
      mask prompts: y0 "Hit crossing offset (y0):"; TOL "Tolerance:"; Ts "Sample time:"
      mask help:
      | The function calculates, using the linear interpolation,an approximation of the time interval error in detencting when the input signal  (y) crosses (in any direction)the offset value "y0".
      | The output (t_err) is the time interval error which value is between 0 and the sample time. The calculation is done (otherwise t_err = 0) if the input signal changes by more then the value defined by the parameter "Tolerance".
      | This change is measured during the time step when the hit crossing takes place.
  gamma_min (deg) : Outport  VectorParamsAs1DForOutWhenUnconnected=off
  gamma_mean (deg) : Outport  Port=2  VectorParamsAs1DForOutWhenUnconnected=off
  Ucom(1-6) : Outport  Port=3  VectorParamsAs1DForOutWhenUnconnected=off
  gamma (deg) : Outport  Port=4  VectorParamsAs1DForOutWhenUnconnected=off
  wires:
  Divide1/1 -> Subtract1/2
  Pulse_counter_sampler (1-6)/2(pulse_n) -> Terminator2/1
  MinMax1/1 -> gamma_min (deg)/1
  Gain1/1 -> gamma_mean (deg)/1
  Sum1/1 -> Gain1/1
  Pulse_counter_sampler (1-6)/1(angle) -> gamma (deg)/1
  Sample and Hold_3/1 -> Product1/1  "t_gamma"
  Subtract1/1 -> Sum/2  "t1"
  Sample and Hold_1/1 -> Sum/1  "t0"
  Gain2/1 -> Product1/2
  Freq/1 -> Gain2/1
  Uabc/1 -> Commutation Voltages/1(Uabc)  "Ua Ub Uc"
  Commutation Voltages/1(Ucom (1-6)) -> Gain7/1, Zero crossing interpolation/1(y), Ucom(1-6)/1
  Gain7/1 -> "Hit (Falling) "/1
  Monostable_1 (4 deg)/1 -> Bistable/1
  "Hit (Falling) "/1 -> Monostable_2 (86 deg)/1
  Sum/1 -> Sample and Hold_3/1
  Product1/1 -> MinMax1/1, Sum1/1, Pulse_counter_sampler (1-6)/1(angles(1-6))  "gamma(1_6)"
  Edge Detector_2/1 -> Sample and Hold_2/2, Sample and Hold_3/2, Zero crossing interpolation/2(Sample)
  Pulses(1-6)/1 -> Pulse_counter_sampler (1-6)/Trigger, Logical Operator2/1
  Logical Operator2/1 -> Logical Operator1/2
  I_th(1-6)/1 -> Hit (Falling)/1
  Logical Operator1/1 -> Monostable_1 (4 deg)/1
  Hit (Falling)/1 -> Logical Operator1/1
  Constant/1 -> Zero crossing interpolation/Enable, Divide1/1
  Clock/1 -> Sample and Hold_2/1, Sample and Hold_1/1
  Zero crossing interpolation/1(t_err) -> Divide1/2  "correction"
  Bistable/1 -> Edge Detector_1/1
  Monostable_2 (86 deg)/1 -> Bistable/2
  Bistable/2 -> Edge Detector_2/1
  Edge Detector_1/1 -> Sample and Hold_1/2
  Sample and Hold_2/1 -> Subtract1/1  "t1_tmp"

== system North_Country_Grid_2024a/Chateauguay HVDC Back-to-Back Converter/Inverter Control and Protection/Inverter Pole Control (Current//Voltage//Gamma)/Alpha Control ==
  note: Alpha Control
  Forced_alpha : Inport
  D_alpha : Inport  Port=2
  Constant1 : Constant  Value=alpha_min
  Constant2 : Constant  Value=alpha_max
  Constant3 : Constant  Value=test_alpha
  Data Type Conversion : DataTypeConversion  OutDataTypeStr=boolean
  Logical Operator : Logic  Operator=OR
  "Rate Limiter (Rate limit) " : RateLimiter  RisingSlewLimit=PRate_fix  FallingSlewLimit=NRate_fix
  "Rate Limiter (Rate limit)    " : RateLimiter  RisingSlewLimit=PRate_fix  FallingSlewLimit=NRate_fix
  Sum : Sum  Inputs=-+  InputSameDT=on  SaturateOnIntegerOverflow=on  OutDataTypeStr=Inherit: Same as first input
  Switch : Switch  Criteria=u2 > Threshold
  Switch1 : Switch  Criteria=u2 > Threshold
  fixed alpha (deg) : Constant  Value=alpha_fix
  Max_i : Outport  VectorParamsAs1DForOutWhenUnconnected=off
  Min_i : Outport  Port=2  VectorParamsAs1DForOutWhenUnconnected=off
  wires:
  "Rate Limiter (Rate limit)    "/1 -> Min_i/1
  "Rate Limiter (Rate limit) "/1 -> Max_i/1
  D_alpha/1 -> Sum/1
  Sum/1 -> Switch/3
  Constant2/1 -> Sum/2
  Constant3/1 -> Logical Operator/1
  Logical Operator/1 -> Switch/2, Switch1/2
  Constant1/1 -> Switch1/3
  Switch/1 -> "Rate Limiter (Rate limit) "/1
  Switch1/1 -> "Rate Limiter (Rate limit)    "/1
  fixed alpha (deg)/1 -> Switch/1, Switch1/1
  Forced_alpha/1 -> Data Type Conversion/1
  Data Type Conversion/1 -> Logical Operator/2

== system North_Country_Grid_2024a/Chateauguay HVDC Back-to-Back Converter/Inverter Control and Protection/Inverter Pole Control (Current//Voltage//Gamma)/Control Mode  ==
  note: AMIN
  note: CONTROL MODE (#):
      |
      | 0) Blocked
      | 1) Current control
      | 2) Voltage control
      | 3) Alpha minimum limitation
      | 4) Alpha maximum limitation
      | 5) Forced or constant Alpha
      | 6) Gamma control
  "a_ord_i " : Inport
  a_ord_v : Inport  Port=2
  a_ord_g : Inport  Port=3
  alpha_ord : Inport  Port=4
  Max_i : Inport  Port=5
  Min_i : Inport  Port=6
  Block : Inport  Port=7
  C : Constant  Value=0
  Data Type Conversion{1..6} (6 alike) : DataTypeConversion  OutDataTypeStr=double  SaturateOnIntegerOverflow=off  RndMeth=Floor
  Gain1 : Gain  Gain=3  OutDataTypeStr=double  SaturateOnIntegerOverflow=on  ParamDataTypeStr=Inherit: Same as input
  Gain2 : Gain  Gain=4  OutDataTypeStr=double  SaturateOnIntegerOverflow=on  ParamDataTypeStr=Inherit: Same as input
  Gain3 : Gain  Gain=2  OutDataTypeStr=double  SaturateOnIntegerOverflow=on  ParamDataTypeStr=Inherit: Same as input
  Gain4 : Gain  Gain=5  OutDataTypeStr=double  SaturateOnIntegerOverflow=on  ParamDataTypeStr=Inherit: Same as input
  Gain5 : Gain  Gain=6  OutDataTypeStr=double  SaturateOnIntegerOverflow=on  ParamDataTypeStr=Inherit: Same as input
  Logical Operator{,1,3,10} (4 alike) : Logic
  Logical Operator2 : Logic  Inputs=3
  Logical Operator4 : Logic  Operator=OR
  Logical Operator{5..7,9} (4 alike) : Logic  Operator=NOT
  Logical Operator8 : Logic  Operator=OR
  MinMax : MinMax  Inputs=2  InputSameDT=on  SaturateOnIntegerOverflow=on
  MinMax1 : MinMax  Inputs=2  InputSameDT=on  SaturateOnIntegerOverflow=on
  Relational Operator : RelationalOperator  Operator=<=
  Relational Operator1 : RelationalOperator  Operator=<=
  Relational Operator2 : RelationalOperator
  Relational Operator3 : RelationalOperator  Operator=<
  Relational Operator4 : RelationalOperator  Operator===
  Sum : Sum  Inputs=++++++  InputSameDT=on  SaturateOnIntegerOverflow=on  OutDataTypeStr=Inherit: Same as first input
  Switch : Switch  Criteria=u2 > Threshold
  mode : Outport  VectorParamsAs1DForOutWhenUnconnected=off
  wires:
  Data Type Conversion6/1 -> Gain4/1
  Data Type Conversion5/1 -> Gain2/1
  Data Type Conversion4/1 -> Gain1/1
  Data Type Conversion3/1 -> Gain5/1
  Data Type Conversion2/1 -> Gain3/1
  Data Type Conversion1/1 -> Sum/1
  Switch/1 -> mode/1
  Logical Operator5/1 -> Logical Operator3/2, Logical Operator/2, Logical Operator10/2
  Logical Operator7/1 -> Logical Operator2/3, Logical Operator1/2
  Gain4/1 -> Sum/5
  Logical Operator1/1 -> Data Type Conversion4/1
  Relational Operator4/1 -> Logical Operator7/1, Data Type Conversion6/1  "AFOR"
  Max_i/1 -> Relational Operator4/2, Relational Operator2/2
  Min_i/1 -> Relational Operator4/1, Relational Operator1/2
  Gain2/1 -> Sum/4
  Gain1/1 -> Sum/3
  Logical Operator2/1 -> Data Type Conversion5/1
  Logical Operator6/1 -> Logical Operator2/1
  Relational Operator2/1 -> Logical Operator2/2, Logical Operator4/2  "AMAX"
  Logical Operator4/1 -> Logical Operator5/1
  Relational Operator1/1 -> Logical Operator1/1, Logical Operator6/1, Logical Operator4/1
  alpha_ord/1 -> Relational Operator2/1, Relational Operator1/1  "alpha_ord"
  Logical Operator/1 -> Data Type Conversion2/1
  Relational Operator3/1 -> Logical Operator/1, Logical Operator8/2  "AVR"
  Gain3/1 -> Sum/2
  Logical Operator3/1 -> Data Type Conversion1/1
  Relational Operator/1 -> Logical Operator3/1, Logical Operator8/1  "ACR"
  "a_ord_i "/1 -> Relational Operator/1, MinMax1/1
  Block/1 -> Switch/2
  Sum/1 -> Switch/3
  C/1 -> Switch/1
  a_ord_v/1 -> MinMax/1, Relational Operator3/1
  a_ord_g/1 -> MinMax/2, MinMax1/2
  MinMax/1 -> Relational Operator/2
  Logical Operator8/1 -> Logical Operator9/1
  Gain5/1 -> Sum/6
  MinMax1/1 -> Relational Operator3/2
  Logical Operator9/1 -> Logical Operator10/1  "AGR"
  Logical Operator10/1 -> Data Type Conversion3/1

== system North_Country_Grid_2024a/Chateauguay HVDC Back-to-Back Converter/Inverter Control and Protection/Inverter Pole Control (Current//Voltage//Gamma)/Current Regulator ==
  note: Current Regulator
  Max_i : Inport
  Min_i : Inport  Port=2
  ERR : Inport  Port=3
  Max_pi : Inport  Port=4
  Min_pi : Inport  Port=5
  Alpha_lin : Inport  Port=6
  Max_lin : Inport  Port=7
  Min_lin : Inport  Port=8
  Inv : Inport  Port=9
  PI Regulator with external limits and linrarized Kp (Discrete) : Subsystem  mask(PI Regulator  With  External  Limits (Discrete)){Kp=Kp_I, Ki=Ki_I, IC_i=ICi_I, On_lin=on, pas=Ts}
      mask prompts: Kp "Kp (deg/pu):"; Ki "Ki (deg/pu/s):"; IC_i "Integrator Initial Condition (deg):"; On_lin "Linearization  (On)"; pas "Sample time (s):"
      mask help: For the linearization it is important to specifie the mode of operation i.e. rectifier or inverter (negation of rectifier).
      mask Display: disp('PI Regulator\nWith external limits\n(Linearized Kp)\n(Discrete)\n\n')
  Alpha_ord : Outport  VectorParamsAs1DForOutWhenUnconnected=off
  wires:
  PI Regulator with external limits and linrarized Kp (Discrete)/1(Alpha_ord) -> Alpha_ord/1
  Max_i/1 -> PI Regulator with external limits and linrarized Kp (Discrete)/1(Max_i)
  Min_i/1 -> PI Regulator with external limits and linrarized Kp (Discrete)/2(Min_i)
  ERR/1 -> PI Regulator with external limits and linrarized Kp (Discrete)/3(ERR)
  Max_pi/1 -> PI Regulator with external limits and linrarized Kp (Discrete)/4(Max_pi)
  Min_pi/1 -> PI Regulator with external limits and linrarized Kp (Discrete)/5(Min_pi)
  Alpha_lin/1 -> PI Regulator with external limits and linrarized Kp (Discrete)/6(Alpha_lin)
  Max_lin/1 -> PI Regulator with external limits and linrarized Kp (Discrete)/7(Max_lin)
  Min_lin/1 -> PI Regulator with external limits and linrarized Kp (Discrete)/8(Min_lin)
  Inv/1 -> PI Regulator with external limits and linrarized Kp (Discrete)/9(Inv)

== system North_Country_Grid_2024a/Chateauguay HVDC Back-to-Back Converter/Inverter Control and Protection/Inverter Pole Control (Current//Voltage//Gamma)/Gamma Error ==
  note: Gamma Error
  G_ref : Inport
  G_meas : Inport  Port=2
  Block : Inport  Port=3
  Id_err : Inport  Port=4
  Enable (Held) : EnablePort  PropagateVarSize=During execution
  Constant1 : Constant  Value=0
  Constant2 : Constant  Value=0
  Constant3 : Constant  Value=G_marg
  Constant4 : Constant  Value=Id_marg
  First-Order Filter (T=0.01) : spsFirstOrderFilterLib/First-Order Filter  FilterType=Lowpass  Tc=0.01  Ts=Ts  Initialize=off  Vac_Init=[0, 0, 60]  Vdc_Init=0  PlotResponse=off  FreqRange="[0,  200,  1]"
  MIN:eps MAX:inf : Saturate  UpperLimit=inf  LowerLimit=eps
  Math Function : Math  Operator=reciprocal  SignedPower=on
  Product1 : Product  Inputs=3  InputSameDT=on  SaturateOnIntegerOverflow=on  OutDataTypeStr=Inherit: Same as first input
  Saturation Dynamic : simulink/Discontinuities/Saturation Dynamic  OutMin=[]  OutMax=[]  OutDataTypeStr=Inherit: Same as second input  OutDataType=fixdt(1, 16)  OutScaling=2^-10  DoSatur=off
  Sum3 : Sum  Inputs=-+-  InputSameDT=on  SaturateOnIntegerOverflow=on  OutDataTypeStr=Inherit: Same as first input
  Switch2 : Switch  Criteria=u2 > Threshold
  ERR_G : Outport  VectorParamsAs1DForOutWhenUnconnected=off
  wires:
  Saturation Dynamic/1 -> Product1/3
  Sum3/1 -> Switch2/3
  G_ref/1 -> Sum3/1
  G_meas/1 -> Sum3/2
  Constant1/1 -> Switch2/1
  Block/1 -> Switch2/2
  Switch2/1 -> ERR_G/1  "ERR"
  Constant2/1 -> Saturation Dynamic/3
  Math Function/1 -> Product1/2
  MIN:eps MAX:inf/1 -> Math Function/1
  Constant4/1 -> MIN:eps MAX:inf/1, Saturation Dynamic/1
  Product1/1 -> First-Order Filter (T=0.01)/1
  First-Order Filter (T=0.01)/1 -> Sum3/3  "dG"
  Id_err/1 -> Saturation Dynamic/2
  Constant3/1 -> Product1/1

== system North_Country_Grid_2024a/Chateauguay HVDC Back-to-Back Converter/Inverter Control and Protection/Inverter Pole Control (Current//Voltage//Gamma)/Gamma Regulator ==
  note: Gamma Regulator
  Max_i : Inport
  Min_i : Inport  Port=2
  ERR : Inport  Port=3
  Max_pi : Inport  Port=4
  Min_pi : Inport  Port=5
  Alpha_lin : Inport  Port=6
  Max_lin : Inport  Port=7
  Min_lin : Inport  Port=8
  Inv : Inport  Port=9
  Enable (Held) : EnablePort  PropagateVarSize=During execution
  PI Regulator with external limits and linrarized Kp (Discrete)1 : Subsystem  mask(PI Regulator  With  External  Limits (Discrete)){Kp=Kp_G, Ki=Ki_G, IC_i=ICi_G, On_lin=on, pas=Ts}
      mask prompts: Kp "Kp (deg/pu):"; Ki "Ki (deg/pu/s):"; IC_i "Integrator Initial Condition (deg):"; On_lin "Linearization  (On)"; pas "Sample time (s):"
      mask help: For the linearization it is important to specifie the mode of operation i.e. rectifier or inverter (negation of rectifier).
      mask Display: disp('PI Regulator\nWith external limits\n(Linearized Kp)\n(Discrete)\n\n')
  Alpha_ord : Outport  VectorParamsAs1DForOutWhenUnconnected=off
  wires:
  PI Regulator with external limits and linrarized Kp (Discrete)1/1(Alpha_ord) -> Alpha_ord/1
  Max_i/1 -> PI Regulator with external limits and linrarized Kp (Discrete)1/1(Max_i)
  Min_i/1 -> PI Regulator with external limits and linrarized Kp (Discrete)1/2(Min_i)
  ERR/1 -> PI Regulator with external limits and linrarized Kp (Discrete)1/3(ERR)
  Max_pi/1 -> PI Regulator with external limits and linrarized Kp (Discrete)1/4(Max_pi)
  Min_pi/1 -> PI Regulator with external limits and linrarized Kp (Discrete)1/5(Min_pi)
  Alpha_lin/1 -> PI Regulator with external limits and linrarized Kp (Discrete)1/6(Alpha_lin)
  Max_lin/1 -> PI Regulator with external limits and linrarized Kp (Discrete)1/7(Max_lin)
  Min_lin/1 -> PI Regulator with external limits and linrarized Kp (Discrete)1/8(Min_lin)
  Inv/1 -> PI Regulator with external limits and linrarized Kp (Discrete)1/9(Inv)
